simulink model "nonlineardtm"  (R2018b)
settings: configuration reference "Physics" (kept outside this file)
model workspace (MAT data in the model file):
  MCOS : class17 (value not decoded)
undefined symbols (not defined in the file): INIT__initialvalues__Vehicle_InitialPitchAngle, INIT__initialvalues__Vehicle_InitialPitchRate_radps, INIT__initialvalues__Vehicle_InitialVelocity_mps__2, INIT__initialvalues__Vehicle_InitialVelocity_mps__3, INIT__initialvalues__Vehicle_InitialYawAngle, INIT__initialvalues__Vehicle_InitialYawRate_radps, tireFL__INERTIAL__m_Wheel_kg, tireFL__SCALING__LCX, tireFL__SCALING__LCY, tireFL__SCALING__LCZ, tireFL__SCALING__LEX, tireFL__SCALING__LEY, tireFL__SCALING__LFZO, tireFL__SCALING__LGAY, tireFL__SCALING__LGAZ, tireFL__SCALING__LHX, tireFL__SCALING__LHY, tireFL__SCALING__LKX, tireFL__SCALING__LKY, tireFL__SCALING__LMPHI, tireFL__SCALING__LMUV, tireFL__SCALING__LMX, tireFL__SCALING__LMY, tireFL__SCALING__LRES, tireFL__SCALING__LS, tireFL__SCALING__LTR, tireFL__SCALING__LVMX, tireFL__SCALING__LVX, tireFL__SCALING__LVY, tireFL__SCALING__LVYKA, tireFL__SCALING__LXAL, tireFL__SCALING__LYKA, tireFR__INERTIAL__m_Wheel_kg, tireFR__SCALING__LCX, tireFR__SCALING__LCY, tireFR__SCALING__LCZ, tireFR__SCALING__LEX, tireFR__SCALING__LEY, tireFR__SCALING__LFZO, tireFR__SCALING__LGAY, tireFR__SCALING__LGAZ, tireFR__SCALING__LHX, tireFR__SCALING__LHY, tireFR__SCALING__LKX, tireFR__SCALING__LKY, tireFR__SCALING__LMPHI, tireFR__SCALING__LMUV, tireFR__SCALING__LMX, tireFR__SCALING__LMY, tireFR__SCALING__LRES, tireFR__SCALING__LS, tireFR__SCALING__LTR, tireFR__SCALING__LVMX, tireFR__SCALING__LVX, tireFR__SCALING__LVY, tireFR__SCALING__LVYKA, tireFR__SCALING__LXAL, tireFR__SCALING__LYKA, tireRL__INERTIAL__m_Wheel_kg, tireRL__SCALING__LCX ... (+71)
libraries: vehdynlibtire_TUM x4, vehdynlibsuspension x2, vrlib x1, vehdynlibeom_TUM x1
(part 4 of 5)

== system nonlineardtm/Nonlinear Dual Track Model/Computation Chassis Coordinate System ==
  TransformationAngles : Inport
  Transformation : Inport  Port=2
  Wheel : Inport  Port=3
  Add : Sum
  Bus Creator : BusCreator  Inputs=10
  Bus Selector2 : BusSelector  OutputSignals=r_I_IRji_m
  Bus Selector3 : BusSelector  OutputSignals=A_F_I
  Bus Selector4 : BusSelector  OutputSignals=chi_IO_rad
  Derivative{,1..3} (4 alike) : Derivative
  Gain : Gain  Gain=1/2
  Gain1 : Gain  Gain=1/2
  Matrix Multiply{,1..3} (4 alike) : Product  Multiplication=Matrix(*)
  Reshape : Reshape  OutputDimensionality=Column vector (2-D)
  Selector : Selector  NumberOfDimensions=2  InputPortWidth=3  IndexOptions=Select all,Index vector (dialog)  Indices=[3 4],[4]  OutputSizes=1,1
  Selector1 : Selector  NumberOfDimensions=2  InputPortWidth=3  IndexOptions=Select all,Index vector (dialog)  Indices=[3 4],[3]  OutputSizes=1,1
  Signal Conversion3 : SignalConversion  OverrideOpt=off
  Signal Specification{,1..9} (10 alike) : SignalSpecification  Dimensions=[3,1]
  Chassis : Outport
  wires:
  Wheel/1 -> Bus Selector2/1
  Transformation/1 -> Bus Selector3/1
  TransformationAngles/1 -> Bus Selector4/1
  Bus Selector4/1 -> Signal Conversion3/1  "<chi_IO_rad>"
  Derivative/1 -> Matrix Multiply2/2, Signal Specification4/1, Derivative1/1
  Derivative1/1 -> Matrix Multiply3/2, Signal Specification5/1
  Signal Conversion3/1 -> Signal Specification3/1, Derivative/1
  Bus Creator/1 -> Chassis/1
  Derivative2/1 -> Matrix Multiply/2, Signal Specification1/1, Derivative3/1
  Bus Selector2/1 -> Selector/1, Selector1/1  "<r_I_IRji_m>"
  Selector/1 -> Gain1/1
  Add/1 -> Reshape/1
  Reshape/1 -> Derivative2/1, Signal Specification/1
  Derivative3/1 -> Matrix Multiply1/2, Signal Specification2/1
  Signal Specification/1 -> Bus Creator/1  "r_I_IF_m"
  Signal Specification1/1 -> Bus Creator/2  "v_I_IF_mps"
  Signal Specification2/1 -> Bus Creator/3  "a_I_IF_mps2"
  Signal Specification3/1 -> Bus Creator/4  "phi_IF_rad"
  Signal Specification4/1 -> Bus Creator/5  "omega_I_IF_radps"
  Signal Specification5/1 -> Bus Creator/6  "alpha_I_IF_radps2"
  Selector1/1 -> Gain/1
  Gain/1 -> Add/1
  Gain1/1 -> Add/2
  Signal Specification6/1 -> Bus Creator/7  "v_F_IF_mps"
  Signal Specification7/1 -> Bus Creator/8  "a_F_IF_mps2"
  Signal Specification8/1 -> Bus Creator/9  "omega_F_IF_radps"
  Signal Specification9/1 -> Bus Creator/10  "alpha_F_IF_radps2"
  Matrix Multiply/1 -> Signal Specification6/1
  Matrix Multiply1/1 -> Signal Specification7/1
  Matrix Multiply2/1 -> Signal Specification8/1
  Matrix Multiply3/1 -> Signal Specification9/1
  Bus Selector3/1 -> Matrix Multiply/1, Matrix Multiply1/1, Matrix Multiply2/1, Matrix Multiply3/1  "<A_F_I>"

== system nonlineardtm/Nonlinear Dual Track Model/Rearrange Force Bus ==
  VehicleForces : Inport
  SuspensionForces : Inport  Port=2
  TireForces : Inport  Port=3
  Bus Creator : BusCreator  Inputs=13
  Bus Selector : BusSelector  OutputSignals=F_K_sum_N,T_K_sum_Nm,F_K_d_N,T_K_d_Nm,F_K_g_N
  Bus Selector1 : BusSelector  OutputSignals=F_K_Aji_N,T_K_Aji_Nm,F_F_Aji_N,T_F_Aji_Nm
  Bus Selector2 : BusSelector  OutputSignals=F_F_Tji_N,T_F_Tji_Nm,F_Tji_Tji_N,T_Tji_Tji_Nm
  Force : Outport
  wires:
  VehicleForces/1 -> Bus Selector/1
  SuspensionForces/1 -> Bus Selector1/1
  TireForces/1 -> Bus Selector2/1
  Bus Selector/1 -> Bus Creator/1  "<F_K_sum_N>"
  Bus Selector2/4 -> Bus Creator/13  "<T_Tji_Tji_Nm>"
  Bus Selector/2 -> Bus Creator/2  "<T_K_sum_Nm>"
  Bus Selector/3 -> Bus Creator/3  "<F_K_d_N>"
  Bus Selector/4 -> Bus Creator/4  "<T_K_d_Nm>"
  Bus Selector/5 -> Bus Creator/5  "<F_K_g_N>"
  Bus Selector1/1 -> Bus Creator/6  "<F_K_Aji_N>"
  Bus Selector1/2 -> Bus Creator/7  "<T_K_Aji_Nm>"
  Bus Selector1/3 -> Bus Creator/8  "<F_F_Aji_N>"
  Bus Selector1/4 -> Bus Creator/9  "<T_F_Aji_Nm>"
  Bus Selector2/1 -> Bus Creator/10  "<F_F_Tji_N>"
  Bus Selector2/2 -> Bus Creator/11  "<T_F_Tji_Nm>"
  Bus Selector2/3 -> Bus Creator/12  "<F_Tji_Tji_N>"
  Bus Creator/1 -> Force/1

== system nonlineardtm/Nonlinear Dual Track Model/Rotation RoadVerticalDisplacement InertialFrame to TireFixed ==
  z_I_Ground_m : Inport
  Gain1 : Gain  Gain=-1
  z_Tji_Ground_m : Outport
  wires:
  Gain1/1 -> z_Tji_Ground_m/1
  z_I_Ground_m/1 -> Gain1/1

== system nonlineardtm/Nonlinear Dual Track Model/Rotation Vertical Position TireFixed to RearAxleFixed z-down ==
  rz_Tji_Rji_m : Inport
  Gain1 : Gain  Gain=-1
  rz_F_Rji_m : Outport
  wires:
  rz_Tji_Rji_m/1 -> Gain1/1
  Gain1/1 -> rz_F_Rji_m/1

== system nonlineardtm/Nonlinear Dual Track Model/Rotation Vertical Velocity TireFixed to RearAxleFixed z-down ==
  vz_Tji_Rji_mps : Inport
  Gain1 : Gain  Gain=-1
  vz_F_Rji_mps : Outport
  wires:
  vz_Tji_Rji_mps/1 -> Gain1/1
  Gain1/1 -> vz_F_Rji_mps/1

== system nonlineardtm/Nonlinear Dual Track Model/Subsystem ==
  r_F_IAji_m : Inport
  v_F_IAji_mps : Inport  Port=2
  delta_ji_rad : Inport  Port=3
  rz_F_IRji_m : Inport  Port=4
  re_Rji_m : Inport  Port=5
  vz_F_IRji_mps : Inport  Port=6
  F_F_Tji_N : Inport  Port=7
  T_F_Tji_Nm : Inport  Port=8
  Selector3 : Selector  NumberOfDimensions=2  InputPortWidth=1  IndexOptions=Index vector (dialog),Select all  Indices=[2],1  OutputSizes=1,1
  Selector38 : Selector  InputPortWidth=4  IndexOptions=Index vector (dialog)  Indices=[1 2]  OutputSizes=1
  Selector6 : Selector  NumberOfDimensions=2  InputPortWidth=1  IndexOptions=Index vector (dialog),Select all  Indices=[1],1  OutputSizes=1,1
  Signal Conversion{1..7,16} (8 alike) : SignalConversion  OverrideOpt=off
  Signal Specification1 : SignalSpecification  Dimensions=[3,4]
  Signal Specification{2,4,6..8} (5 alike) : SignalSpecification  Dimensions=[1,4]
  Signal Specification3 : SignalSpecification  Dimensions=[3,4]
  Signal Specification5 : SignalSpecification  Dimensions=[3,4]
  VehP [3x4] : Outport
  VehV [3x4] : Outport  Port=2
  StrgAngF [1x2] : Outport  Port=3
  WhlPz [1x4] : Outport  Port=4
  WhlRe [1x4] : Outport  Port=5
  WhlVz [1x4] : Outport  Port=6
  WhlFx [1x4] : Outport  Port=7
  WhlFy [1x4] : Outport  Port=8
  WhlM [3x4] : Outport  Port=9
  wires:
  r_F_IAji_m/1 -> Signal Conversion16/1
  v_F_IAji_mps/1 -> Signal Conversion1/1
  delta_ji_rad/1 -> Signal Conversion2/1
  Signal Specification3/1 -> VehP [3x4]/1
  Signal Specification1/1 -> VehV [3x4]/1
  F_F_Tji_N/1 -> Signal Conversion6/1
  Selector6/1 -> Signal Specification2/1
  Selector3/1 -> Signal Specification4/1
  Signal Specification2/1 -> WhlFx [1x4]/1
  Signal Specification4/1 -> WhlFy [1x4]/1
  Selector38/1 -> StrgAngF [1x2]/1
  T_F_Tji_Nm/1 -> Signal Conversion7/1
  Signal Specification5/1 -> WhlM [3x4]/1
  Signal Specification8/1 -> WhlPz [1x4]/1
  Signal Specification7/1 -> WhlRe [1x4]/1
  Signal Specification6/1 -> WhlVz [1x4]/1
  vz_F_IRji_mps/1 -> Signal Conversion5/1
  re_Rji_m/1 -> Signal Conversion4/1
  rz_F_IRji_m/1 -> Signal Conversion3/1
  Signal Conversion16/1 -> Signal Specification3/1
  Signal Conversion1/1 -> Signal Specification1/1
  Signal Conversion2/1 -> Selector38/1
  Signal Conversion3/1 -> Signal Specification8/1
  Signal Conversion4/1 -> Signal Specification7/1
  Signal Conversion5/1 -> Signal Specification6/1
  Signal Conversion7/1 -> Signal Specification5/1
  Signal Conversion6/1 -> Selector3/1, Selector6/1

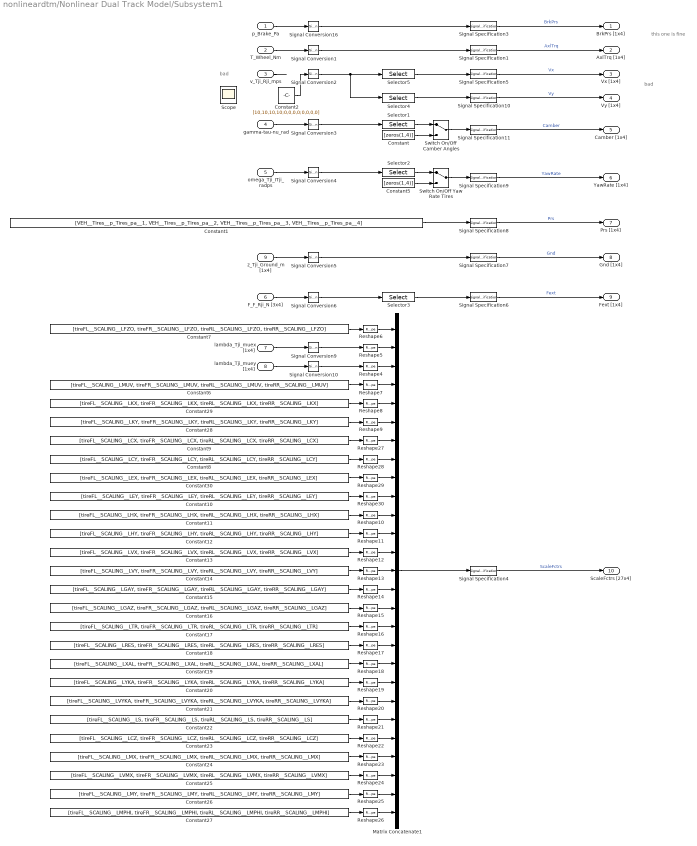
== system nonlineardtm/Nonlinear Dual Track Model/Subsystem1 ==
  note: bad
  note: bad
  note: this one is fine
  p_Brake_Pa : Inport
  T_Wheel_Nm : Inport  Port=2
  v_Tji_Rji_mps : Inport  Port=3
  gamma-tau-nu_rad : Inport  Port=4
  omega_Tji_ITji_radps : Inport  Port=5
  F_F_Rji_N [3x4] : Inport  Port=6
  lambda_Tji_muex [1x4] : Inport  Port=7
  lambda_Tji_muey [1x4] : Inport  Port=8
  z_Tji_Ground_m [1x4] : Inport  Port=9
  Constant : Constant  Value=[zeros(1,4)]
  Constant1 : Constant  Value=[VEH__Tires__p_Tires_pa__1, VEH__Tires__p_Tires_pa__2, VEH__Tires__p_Tires_pa__3, VEH__Tires__p_Tires_pa__4]
  Constant10 : Constant  Value=[tireFL__SCALING__LEY, tireFR__SCALING__LEY, tireRL__SCALING__LEY, tireRR__SCALING__LEY]
  Constant11 : Constant  Value=[tireFL__SCALING__LHX, tireFR__SCALING__LHX, tireRL__SCALING__LHX, tireRR__SCALING__LHX]
  Constant12 : Constant  Value=[tireFL__SCALING__LHY, tireFR__SCALING__LHY, tireRL__SCALING__LHY, tireRR__SCALING__LHY]
  Constant13 : Constant  Value=[tireFL__SCALING__LVX, tireFR__SCALING__LVX, tireRL__SCALING__LVX, tireRR__SCALING__LVX]
  Constant14 : Constant  Value=[tireFL__SCALING__LVY, tireFR__SCALING__LVY, tireRL__SCALING__LVY, tireRR__SCALING__LVY]
  Constant15 : Constant  Value=[tireFL__SCALING__LGAY, tireFR__SCALING__LGAY, tireRL__SCALING__LGAY, tireRR__SCALING__LGAY]
  Constant16 : Constant  Value=[tireFL__SCALING__LGAZ, tireFR__SCALING__LGAZ, tireRL__SCALING__LGAZ, tireRR__SCALING__LGAZ]
  Constant17 : Constant  Value=[tireFL__SCALING__LTR, tireFR__SCALING__LTR, tireRL__SCALING__LTR, tireRR__SCALING__LTR]
  Constant18 : Constant  Value=[tireFL__SCALING__LRES, tireFR__SCALING__LRES, tireRL__SCALING__LRES, tireRR__SCALING__LRES]
  Constant19 : Constant  Value=[tireFL__SCALING__LXAL, tireFR__SCALING__LXAL, tireRL__SCALING__LXAL, tireRR__SCALING__LXAL]
  Constant2 : Constant  Value=[10,10,10,10;0,0,0,0;0,0,0,0]  VectorParams1D=off
  Constant20 : Constant  Value=[tireFL__SCALING__LYKA, tireFR__SCALING__LYKA, tireRL__SCALING__LYKA, tireRR__SCALING__LYKA]
  Constant21 : Constant  Value=[tireFL__SCALING__LVYKA, tireFR__SCALING__LVYKA, tireRL__SCALING__LVYKA, tireRR__SCALING__LVYKA]
  Constant22 : Constant  Value=[tireFL__SCALING__LS, tireFR__SCALING__LS, tireRL__SCALING__LS, tireRR__SCALING__LS]
  Constant23 : Constant  Value=[tireFL__SCALING__LCZ, tireFR__SCALING__LCZ, tireRL__SCALING__LCZ, tireRR__SCALING__LCZ]
  Constant24 : Constant  Value=[tireFL__SCALING__LMX, tireFR__SCALING__LMX, tireRL__SCALING__LMX, tireRR__SCALING__LMX]
  Constant25 : Constant  Value=[tireFL__SCALING__LVMX, tireFR__SCALING__LVMX, tireRL__SCALING__LVMX, tireRR__SCALING__LVMX]
  Constant26 : Constant  Value=[tireFL__SCALING__LMY, tireFR__SCALING__LMY, tireRL__SCALING__LMY, tireRR__SCALING__LMY]
  Constant27 : Constant  Value=[tireFL__SCALING__LMPHI, tireFR__SCALING__LMPHI, tireRL__SCALING__LMPHI, tireRR__SCALING__LMPHI]
  Constant28 : Constant  Value=[tireFL__SCALING__LKY, tireFR__SCALING__LKY, tireRL__SCALING__LKY, tireRR__SCALING__LKY]
  Constant29 : Constant  Value=[tireFL__SCALING__LKX, tireFR__SCALING__LKX, tireRL__SCALING__LKX, tireRR__SCALING__LKX]
  Constant30 : Constant  Value=[tireFL__SCALING__LEX, tireFR__SCALING__LEX, tireRL__SCALING__LEX, tireRR__SCALING__LEX]
  Constant5 : Constant  Value=[zeros(1,4)]
  Constant6 : Constant  Value=[tireFL__SCALING__LMUV, tireFR__SCALING__LMUV, tireRL__SCALING__LMUV, tireRR__SCALING__LMUV]
  Constant7 : Constant  Value=[tireFL__SCALING__LFZO, tireFR__SCALING__LFZO, tireRL__SCALING__LFZO, tireRR__SCALING__LFZO]
  Constant8 : Constant  Value=[tireFL__SCALING__LCY, tireFR__SCALING__LCY, tireRL__SCALING__LCY, tireRR__SCALING__LCY]
  Constant9 : Constant  Value=[tireFL__SCALING__LCX, tireFR__SCALING__LCX, tireRL__SCALING__LCX, tireRR__SCALING__LCX]
  Matrix Concatenate1 : Concatenate  NumInputs=27  Mode=Multidimensional array
  Reshape{4..30} (27 alike) : Reshape  OutputDimensionality=Row vector (2-D)
  Scope : Scope
  Selector1 : Selector  NumberOfDimensions=2  InputPortWidth=3  IndexOptions=Index vector (dialog),Select all  Indices=1,1  OutputSizes=1,1
  Selector2 : Selector  NumberOfDimensions=2  InputPortWidth=3  IndexOptions=Index vector (dialog),Select all  Indices=3,1  OutputSizes=1,1
  Selector3 : Selector  NumberOfDimensions=2  InputPortWidth=3  IndexOptions=Index vector (dialog),Select all  Indices=3,1  OutputSizes=1,1
  Selector4 : Selector  NumberOfDimensions=2  InputPortWidth=1  IndexOptions=Index vector (dialog),Select all  Indices=[2],1  OutputSizes=1,1
  Selector5 : Selector  NumberOfDimensions=2  InputPortWidth=1  IndexOptions=Index vector (dialog),Select all  Indices=[1],1  OutputSizes=1,1
  Signal Conversion{1..6,9..10,16} (9 alike) : SignalConversion  OverrideOpt=off
  Signal Specification{1,3,5..11} (9 alike) : SignalSpecification  Dimensions=[1,4]
  Signal Specification4 : SignalSpecification  Dimensions=[27,4]
  Switch On/Off Camber Angles : ManualSwitch
  Switch On/Off Yaw Rate Tires : ManualSwitch
  BrkPrs [1x4] : Outport
  AxlTrq [1x4] : Outport  Port=2
  Vx [1x4] : Outport  Port=3
  Vy [1x4] : Outport  Port=4
  Camber [1x4] : Outport  Port=5
  YawRate [1x4] : Outport  Port=6
  Prs [1x4] : Outport  Port=7
  Gnd [1x4] : Outport  Port=8
  Fext [1x4] : Outport  Port=9
  ScaleFctrs [27x4] : Outport  Port=10
  wires:
  Signal Specification9/1 -> YawRate [1x4]/1  "YawRate"
  Signal Specification1/1 -> AxlTrq [1x4]/1  "AxlTrq"
  Signal Specification4/1 -> ScaleFctrs [27x4]/1  "ScaleFctrs"
  Signal Specification8/1 -> Prs [1x4]/1  "Prs"
  Signal Specification7/1 -> Gnd [1x4]/1  "Gnd"
  Signal Specification6/1 -> Fext [1x4]/1  "Fext"
  Signal Specification5/1 -> Vx [1x4]/1  "Vx"
  Signal Specification10/1 -> Vy [1x4]/1  "Vy"
  Constant1/1 -> Signal Specification8/1
  Signal Specification11/1 -> Camber [1x4]/1  "Camber"
  Selector1/1 -> Switch On/Off Camber Angles/1
  Switch On/Off Camber Angles/1 -> Signal Specification11/1
  Constant/1 -> Switch On/Off Camber Angles/2
  Constant5/1 -> Switch On/Off Yaw Rate Tires/2
  Switch On/Off Yaw Rate Tires/1 -> Signal Specification9/1
  Selector2/1 -> Switch On/Off Yaw Rate Tires/1
  p_Brake_Pa/1 -> Signal Conversion16/1
  T_Wheel_Nm/1 -> Signal Conversion1/1
  gamma-tau-nu_rad/1 -> Signal Conversion3/1
  omega_Tji_ITji_radps/1 -> Signal Conversion4/1
  z_Tji_Ground_m [1x4]/1 -> Signal Conversion5/1
  F_F_Rji_N [3x4]/1 -> Signal Conversion6/1
  Signal Specification3/1 -> BrkPrs [1x4]/1  "BrkPrs"
  Signal Conversion16/1 -> Signal Specification3/1
  Signal Conversion1/1 -> Signal Specification1/1
  Signal Conversion3/1 -> Selector1/1
  Signal Conversion5/1 -> Signal Specification7/1
  Signal Conversion2/1 -> Selector4/1, Selector5/1
  Signal Conversion4/1 -> Selector2/1
  Signal Conversion6/1 -> Selector3/1
  Selector5/1 -> Signal Specification5/1
  Selector4/1 -> Signal Specification10/1
  Selector3/1 -> Signal Specification6/1
  lambda_Tji_muey [1x4]/1 -> Signal Conversion10/1
  lambda_Tji_muex [1x4]/1 -> Signal Conversion9/1
  Constant7/1 -> Reshape6/1
  Reshape5/1 -> Matrix Concatenate1/2
  Reshape27/1 -> Matrix Concatenate1/7
  Constant28/1 -> Reshape9/1
  Constant13/1 -> Reshape12/1
  Constant9/1 -> Reshape27/1
  Reshape7/1 -> Matrix Concatenate1/4
  Reshape16/1 -> Matrix Concatenate1/17
  Constant21/1 -> Reshape20/1
  Reshape11/1 -> Matrix Concatenate1/12
  Reshape9/1 -> Matrix Concatenate1/6
  Signal Conversion9/1 -> Reshape5/1
  Reshape17/1 -> Matrix Concatenate1/18
  Reshape25/1 -> Matrix Concatenate1/26
  Reshape29/1 -> Matrix Concatenate1/9
  Constant29/1 -> Reshape8/1
  Constant12/1 -> Reshape11/1
  Constant30/1 -> Reshape29/1
  Signal Conversion10/1 -> Reshape4/1
  Reshape24/1 -> Matrix Concatenate1/25
  Constant20/1 -> Reshape19/1
  Constant6/1 -> Reshape7/1
  Constant15/1 -> Reshape14/1
  Constant26/1 -> Reshape25/1
  Reshape12/1 -> Matrix Concatenate1/13
  Constant11/1 -> Reshape10/1
  Constant16/1 -> Reshape15/1
  Constant23/1 -> Reshape22/1
  Reshape15/1 -> Matrix Concatenate1/16
  Reshape10/1 -> Matrix Concatenate1/11
  Reshape18/1 -> Matrix Concatenate1/19
  Matrix Concatenate1/1 -> Signal Specification4/1
  Constant22/1 -> Reshape21/1
  Reshape6/1 -> Matrix Concatenate1/1
  Constant10/1 -> Reshape30/1
  Reshape26/1 -> Matrix Concatenate1/27
  Reshape14/1 -> Matrix Concatenate1/15
  Reshape4/1 -> Matrix Concatenate1/3
  Reshape22/1 -> Matrix Concatenate1/23
  Reshape20/1 -> Matrix Concatenate1/21
  Constant19/1 -> Reshape18/1
  Reshape8/1 -> Matrix Concatenate1/5
  Constant18/1 -> Reshape17/1
  Constant17/1 -> Reshape16/1
  Reshape19/1 -> Matrix Concatenate1/20
  Reshape30/1 -> Matrix Concatenate1/10
  Constant27/1 -> Reshape26/1
  Reshape13/1 -> Matrix Concatenate1/14
  Reshape21/1 -> Matrix Concatenate1/22
  Constant14/1 -> Reshape13/1
  Reshape28/1 -> Matrix Concatenate1/8
  Reshape23/1 -> Matrix Concatenate1/24
  Constant24/1 -> Reshape23/1
  Constant25/1 -> Reshape24/1
  Constant8/1 -> Reshape28/1
  v_Tji_Rji_mps/1 -> ?
  Constant2/1 -> Signal Conversion2/1

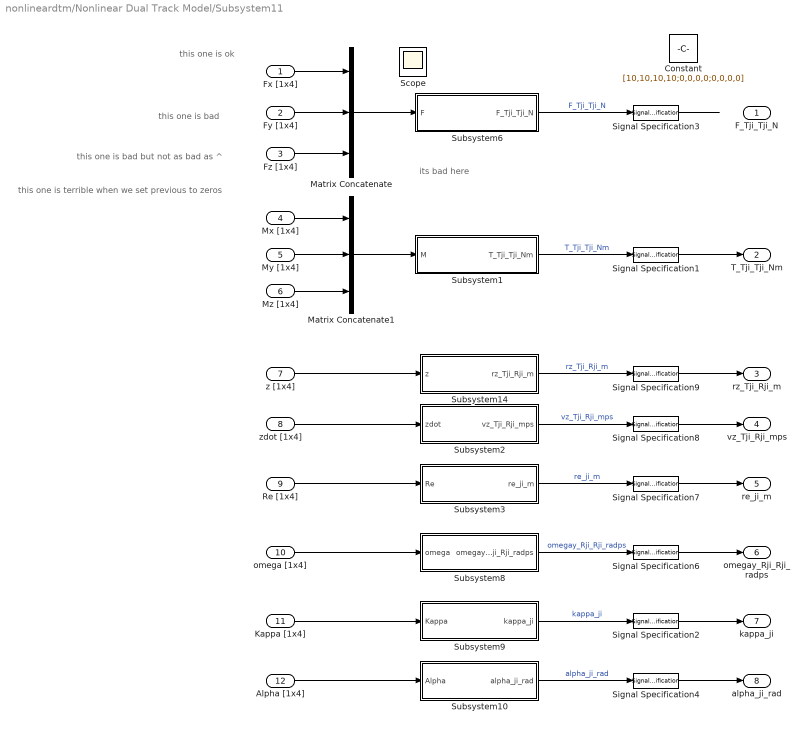
== system nonlineardtm/Nonlinear Dual Track Model/Subsystem11 ==
  note: this one is terrible when we set previous to zeros
  note: this one is bad but not as bad as ^
  note: this one is bad
  note: its bad here
  note: this one is ok
  Fx [1x4] : Inport
  Fy [1x4] : Inport  Port=2
  Fz [1x4] : Inport  Port=3
  Mx [1x4] : Inport  Port=4
  My [1x4] : Inport  Port=5
  Mz [1x4] : Inport  Port=6
  z [1x4] : Inport  Port=7
  zdot [1x4] : Inport  Port=8
  Re [1x4] : Inport  Port=9
  omega [1x4] : Inport  Port=10
  Kappa [1x4] : Inport  Port=11
  Alpha [1x4] : Inport  Port=12
  Constant : Constant  Value=[10,10,10,10;0,0,0,0;0,0,0,0]
  Matrix Concatenate : Concatenate  NumInputs=3  Mode=Multidimensional array
  Matrix Concatenate1 : Concatenate  NumInputs=3  Mode=Multidimensional array
  Scope : Scope
  Signal Specification1 : SignalSpecification  Dimensions=[3,4]
  Signal Specification{2,4,6..9} (6 alike) : SignalSpecification  Dimensions=[1,4]
  Signal Specification3 : SignalSpecification  Dimensions=[3,4]
  Subsystem1 : Subsystem
  Subsystem10 : Subsystem
  Subsystem14 : Subsystem
  Subsystem2 : Subsystem
  Subsystem3 : Subsystem
  Subsystem6 : Subsystem
  Subsystem8 : Subsystem
  Subsystem9 : Subsystem
  F_Tji_Tji_N : Outport
  T_Tji_Tji_Nm : Outport  Port=2
  rz_Tji_Rji_m : Outport  Port=3
  vz_Tji_Rji_mps : Outport  Port=4
  re_ji_m : Outport  Port=5
  omegay_Rji_Rji_radps : Outport  Port=6
  kappa_ji : Outport  Port=7
  alpha_ji_rad : Outport  Port=8
  wires:
  Signal Specification6/1 -> omegay_Rji_Rji_radps/1
  Signal Specification7/1 -> re_ji_m/1
  Signal Specification8/1 -> vz_Tji_Rji_mps/1
  Signal Specification4/1 -> alpha_ji_rad/1
  Signal Specification2/1 -> kappa_ji/1
  Signal Specification1/1 -> T_Tji_Tji_Nm/1
  Signal Specification3/1 -> ?
  Mx [1x4]/1 -> Matrix Concatenate1/1
  Subsystem14/1(rz_Tji_Rji_m) -> Signal Specification9/1  "rz_Tji_Rji_m"
  Fz [1x4]/1 -> Matrix Concatenate/3
  Mz [1x4]/1 -> Matrix Concatenate1/3
  My [1x4]/1 -> Matrix Concatenate1/2
  Fy [1x4]/1 -> Matrix Concatenate/2
  Fx [1x4]/1 -> Matrix Concatenate/1
  Signal Specification9/1 -> rz_Tji_Rji_m/1
  z [1x4]/1 -> Subsystem14/1(z)
  zdot [1x4]/1 -> Subsystem2/1(zdot)
  Re [1x4]/1 -> Subsystem3/1(Re)
  omega [1x4]/1 -> Subsystem8/1(omega)
  Kappa [1x4]/1 -> Subsystem9/1(Kappa)
  Alpha [1x4]/1 -> Subsystem10/1(Alpha)
  Subsystem2/1(vz_Tji_Rji_mps) -> Signal Specification8/1  "vz_Tji_Rji_mps"
  Subsystem3/1(re_ji_m) -> Signal Specification7/1  "re_ji_m"
  Subsystem8/1(omegay_Rji_Rji_radps) -> Signal Specification6/1  "omegay_Rji_Rji_radps"
  Subsystem9/1(kappa_ji) -> Signal Specification2/1  "kappa_ji"
  Subsystem10/1(alpha_ji_rad) -> Signal Specification4/1  "alpha_ji_rad"
  Subsystem1/1(T_Tji_Tji_Nm) -> Signal Specification1/1  "T_Tji_Tji_Nm"
  Subsystem6/1(F_Tji_Tji_N) -> Signal Specification3/1  "F_Tji_Tji_N"
  Matrix Concatenate1/1 -> Subsystem1/1(M)
  Matrix Concatenate/1 -> Subsystem6/1(F)

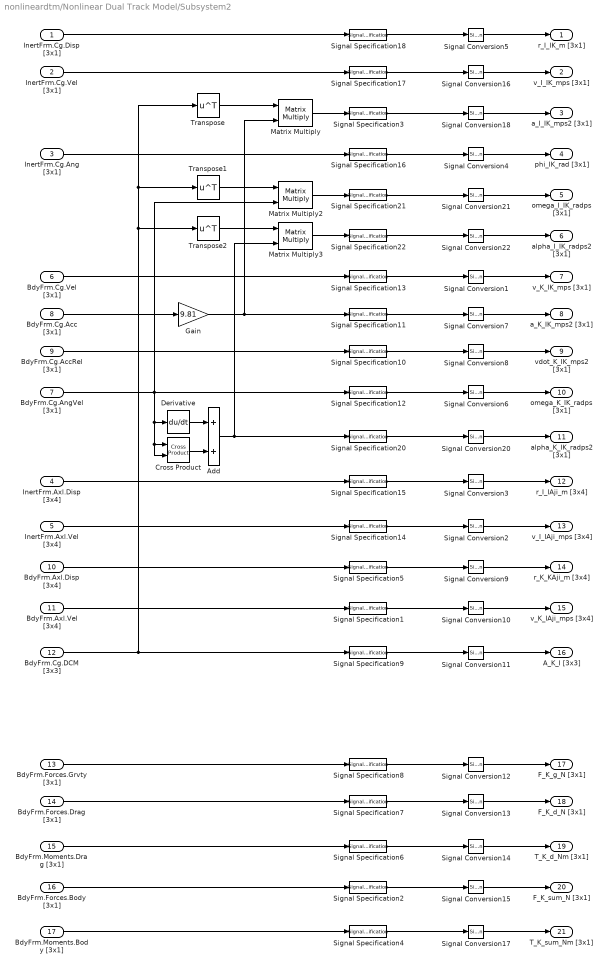
== system nonlineardtm/Nonlinear Dual Track Model/Subsystem2 ==
  InertFrm.Cg.Disp [3x1] : Inport
  InertFrm.Cg.Vel [3x1] : Inport  Port=2
  InertFrm.Cg.Ang [3x1] : Inport  Port=3
  InertFrm.Axl.Disp [3x4] : Inport  Port=4
  InertFrm.Axl.Vel [3x4] : Inport  Port=5
  BdyFrm.Cg.Vel [3x1] : Inport  Port=6
  BdyFrm.Cg.AngVel [3x1] : Inport  Port=7
  BdyFrm.Cg.Acc [3x1] : Inport  Port=8
  BdyFrm.Cg.AccRel [3x1] : Inport  Port=9
  BdyFrm.Axl.Disp [3x4] : Inport  Port=10
  BdyFrm.Axl.Vel [3x4] : Inport  Port=11
  BdyFrm.Cg.DCM [3x3] : Inport  Port=12
  BdyFrm.Forces.Grvty [3x1] : Inport  Port=13
  BdyFrm.Forces.Drag [3x1] : Inport  Port=14
  BdyFrm.Moments.Drag [3x1] : Inport  Port=15
  BdyFrm.Forces.Body [3x1] : Inport  Port=16
  BdyFrm.Moments.Body [3x1] : Inport  Port=17
  Add : Sum
  Cross Product : vrlib/Utilities/Cross Product
      settings: SourceProductBaseCode=VR
  Derivative : Derivative
  Gain : Gain  Gain=9.81
  Matrix Multiply : Product  Multiplication=Matrix(*)
  Matrix Multiply2 : Product  Multiplication=Matrix(*)
  Matrix Multiply3 : Product  Multiplication=Matrix(*)
  Signal Conversion{1..18,20..22} (21 alike) : SignalConversion  OverrideOpt=off
  Signal Specification{1,5,14..15} (4 alike) : SignalSpecification  Dimensions=[3,4]
  Signal Specification{2..4,6..8,10..13,16..18,20..22} (16 alike) : SignalSpecification  Dimensions=[3,1]
  Signal Specification9 : SignalSpecification  Dimensions=[3,3]
  Transpose : Math  Operator=transpose  SaturateOnIntegerOverflow=on
  Transpose1 : Math  Operator=transpose  SaturateOnIntegerOverflow=on
  Transpose2 : Math  Operator=transpose  SaturateOnIntegerOverflow=on
  r_I_IK_m [3x1] : Outport
  v_I_IK_mps [3x1] : Outport  Port=2
  a_I_IK_mps2 [3x1] : Outport  Port=3
  phi_IK_rad [3x1] : Outport  Port=4
  omega_I_IK_radps [3x1] : Outport  Port=5
  alpha_I_IK_radps2 [3x1] : Outport  Port=6
  v_K_IK_mps [3x1] : Outport  Port=7
  a_K_IK_mps2 [3x1] : Outport  Port=8
  vdot_K_IK_mps2 [3x1] : Outport  Port=9
  omega_K_IK_radps [3x1] : Outport  Port=10
  alpha_K_IK_radps2 [3x1] : Outport  Port=11
  r_I_IAji_m [3x4] : Outport  Port=12
  v_I_IAji_mps [3x4] : Outport  Port=13
  r_K_KAji_m [3x4] : Outport  Port=14
  v_K_IAji_mps [3x4] : Outport  Port=15
  A_K_I [3x3] : Outport  Port=16
  F_K_g_N [3x1] : Outport  Port=17
  F_K_d_N [3x1] : Outport  Port=18
  T_K_d_Nm [3x1] : Outport  Port=19
  F_K_sum_N [3x1] : Outport  Port=20
  T_K_sum_Nm [3x1] : Outport  Port=21
  wires:
  Signal Specification5/1 -> Signal Conversion9/1
  Signal Specification11/1 -> Signal Conversion7/1
  Signal Specification7/1 -> Signal Conversion13/1
  Signal Specification16/1 -> Signal Conversion4/1
  Signal Specification8/1 -> Signal Conversion12/1
  Signal Specification6/1 -> Signal Conversion14/1
  Signal Specification12/1 -> Signal Conversion6/1
  Signal Specification1/1 -> Signal Conversion10/1
  Signal Specification9/1 -> Signal Conversion11/1
  Signal Specification15/1 -> Signal Conversion3/1
  Signal Specification18/1 -> Signal Conversion5/1
  Signal Specification4/1 -> Signal Conversion17/1
  Signal Specification13/1 -> Signal Conversion1/1
  Signal Specification10/1 -> Signal Conversion8/1
  Signal Specification14/1 -> Signal Conversion2/1
  Signal Specification2/1 -> Signal Conversion15/1
  Signal Specification17/1 -> Signal Conversion16/1
  BdyFrm.Cg.Acc [3x1]/1 -> Gain/1
  InertFrm.Cg.Disp [3x1]/1 -> Signal Specification18/1
  InertFrm.Cg.Vel [3x1]/1 -> Signal Specification17/1
  InertFrm.Cg.Ang [3x1]/1 -> Signal Specification16/1
  InertFrm.Axl.Disp [3x4]/1 -> Signal Specification15/1
  InertFrm.Axl.Vel [3x4]/1 -> Signal Specification14/1
  BdyFrm.Cg.Vel [3x1]/1 -> Signal Specification13/1
  BdyFrm.Cg.AngVel [3x1]/1 -> Cross Product/2, Cross Product/1, Derivative/1, Matrix Multiply2/2, Signal Specification12/1
  Gain/1 -> Signal Specification11/1, Matrix Multiply/2
  BdyFrm.Cg.AccRel [3x1]/1 -> Signal Specification10/1
  BdyFrm.Axl.Disp [3x4]/1 -> Signal Specification5/1
  BdyFrm.Axl.Vel [3x4]/1 -> Signal Specification1/1
  BdyFrm.Cg.DCM [3x3]/1 -> Signal Specification9/1, Transpose1/1, Transpose/1, Transpose2/1
  BdyFrm.Forces.Grvty [3x1]/1 -> Signal Specification8/1
  BdyFrm.Forces.Drag [3x1]/1 -> Signal Specification7/1
  BdyFrm.Moments.Drag [3x1]/1 -> Signal Specification6/1
  BdyFrm.Forces.Body [3x1]/1 -> Signal Specification2/1
  BdyFrm.Moments.Body [3x1]/1 -> Signal Specification4/1
  Signal Conversion16/1 -> v_I_IK_mps [3x1]/1
  Signal Conversion5/1 -> r_I_IK_m [3x1]/1
  Signal Conversion4/1 -> phi_IK_rad [3x1]/1
  Signal Conversion3/1 -> r_I_IAji_m [3x4]/1
  Signal Conversion2/1 -> v_I_IAji_mps [3x4]/1
  Signal Conversion1/1 -> v_K_IK_mps [3x1]/1
  Signal Conversion6/1 -> omega_K_IK_radps [3x1]/1
  Signal Conversion7/1 -> a_K_IK_mps2 [3x1]/1
  Signal Conversion8/1 -> vdot_K_IK_mps2 [3x1]/1
  Signal Conversion9/1 -> r_K_KAji_m [3x4]/1
  Signal Conversion10/1 -> v_K_IAji_mps [3x4]/1
  Signal Conversion11/1 -> A_K_I [3x3]/1
  Signal Conversion12/1 -> F_K_g_N [3x1]/1
  Signal Conversion13/1 -> F_K_d_N [3x1]/1
  Signal Conversion14/1 -> T_K_d_Nm [3x1]/1
  Signal Conversion15/1 -> F_K_sum_N [3x1]/1
  Signal Conversion17/1 -> T_K_sum_Nm [3x1]/1
  Signal Conversion18/1 -> a_I_IK_mps2 [3x1]/1
  Signal Specification3/1 -> Signal Conversion18/1
  Matrix Multiply/1 -> Signal Specification3/1
  Transpose/1 -> Matrix Multiply/1
  Signal Conversion20/1 -> alpha_K_IK_radps2 [3x1]/1
  Signal Specification20/1 -> Signal Conversion20/1
  Derivative/1 -> Add/1
  Add/1 -> Signal Specification20/1, Matrix Multiply3/2
  Cross Product/1 -> Add/2
  Signal Conversion21/1 -> omega_I_IK_radps [3x1]/1
  Signal Specification21/1 -> Signal Conversion21/1
  Matrix Multiply2/1 -> Signal Specification21/1
  Transpose1/1 -> Matrix Multiply2/1
  Matrix Multiply3/1 -> Signal Specification22/1
  Signal Specification22/1 -> Signal Conversion22/1
  Signal Conversion22/1 -> alpha_I_IK_radps2 [3x1]/1
  Transpose2/1 -> Matrix Multiply3/1

== system nonlineardtm/Nonlinear Dual Track Model/Subsystem3 ==
  F_K_Extern_N : Inport
  T_K_Extern_Nm : Inport  Port=2
  v_I_Wind_mps : Inport  Port=3
  F_K_Aji_N : Inport  Port=4
  T_K_Aji_Nm : Inport  Port=5
  Signal Conversion{1..4,16} (5 alike) : SignalConversion  OverrideOpt=off
  Signal Specification1 : SignalSpecification  Dimensions=[3,1]
  Signal Specification2 : SignalSpecification  Dimensions=[3,1]
  Signal Specification3 : SignalSpecification  Dimensions=[3,1]
  Signal Specification7 : SignalSpecification  Dimensions=[3,4]
  Signal Specification8 : SignalSpecification  Dimensions=[3,4]
  FExt [3x1] : Outport
  MExt [3x1] : Outport  Port=2
  WindXYZ [3x1] : Outport  Port=3
  FSusp [3x4] : Outport  Port=4
  MSusp [3x4] : Outport  Port=5
  wires:
  v_I_Wind_mps/1 -> Signal Specification2/1
  Signal Specification2/1 -> Signal Conversion2/1
  T_K_Aji_Nm/1 -> Signal Specification8/1
  F_K_Aji_N/1 -> Signal Specification7/1
  T_K_Extern_Nm/1 -> Signal Specification1/1
  F_K_Extern_N/1 -> Signal Specification3/1
  Signal Conversion4/1 -> MSusp [3x4]/1
  Signal Conversion3/1 -> FSusp [3x4]/1
  Signal Conversion1/1 -> MExt [3x1]/1
  Signal Conversion16/1 -> FExt [3x1]/1
  Signal Specification7/1 -> Signal Conversion3/1
  Signal Specification8/1 -> Signal Conversion4/1
  Signal Conversion2/1 -> WindXYZ [3x1]/1
  Signal Specification1/1 -> Signal Conversion1/1
  Signal Specification3/1 -> Signal Conversion16/1

== system nonlineardtm/Nonlinear Dual Track Model/Subsystem4 ==
  VehF [3x4] : Inport
  VehM [3x4] : Inport  Port=2
  WhlF [3x4] : Inport  Port=3
  WhlV [3x4] : Inport  Port=4
  WhlAng [3x4] : Inport  Port=5
  SuspH [1x4] : Inport  Port=6
  Signal Conversion{1..5,16} (6 alike) : SignalConversion  OverrideOpt=off
  Signal Specification{1..5} (5 alike) : SignalSpecification  Dimensions=[3,4]
  Signal Specification6 : SignalSpecification  Dimensions=[1,4]
  F_F_Aji_N : Outport
  T_F_Aji_Nm : Outport  Port=2
  F_F_Rji_N : Outport  Port=3
  v_F_IRji_mps : Outport  Port=4
  gamma-tau-nu_rad : Outport  Port=5
  h_ji_m : Outport  Port=6
  wires:
  Signal Specification3/1 -> F_F_Aji_N/1
  Signal Specification1/1 -> T_F_Aji_Nm/1
  WhlF [3x4]/1 -> Signal Conversion2/1
  Signal Specification4/1 -> v_F_IRji_mps/1
  Signal Specification5/1 -> gamma-tau-nu_rad/1
  Signal Specification6/1 -> h_ji_m/1
  VehF [3x4]/1 -> Signal Conversion16/1
  VehM [3x4]/1 -> Signal Conversion1/1
  WhlV [3x4]/1 -> Signal Conversion3/1
  WhlAng [3x4]/1 -> Signal Conversion4/1
  SuspH [1x4]/1 -> Signal Conversion5/1
  Signal Specification2/1 -> F_F_Rji_N/1
  Signal Conversion16/1 -> Signal Specification3/1
  Signal Conversion1/1 -> Signal Specification1/1
  Signal Conversion2/1 -> Signal Specification2/1
  Signal Conversion3/1 -> Signal Specification4/1
  Signal Conversion4/1 -> Signal Specification5/1
  Signal Conversion5/1 -> Signal Specification6/1

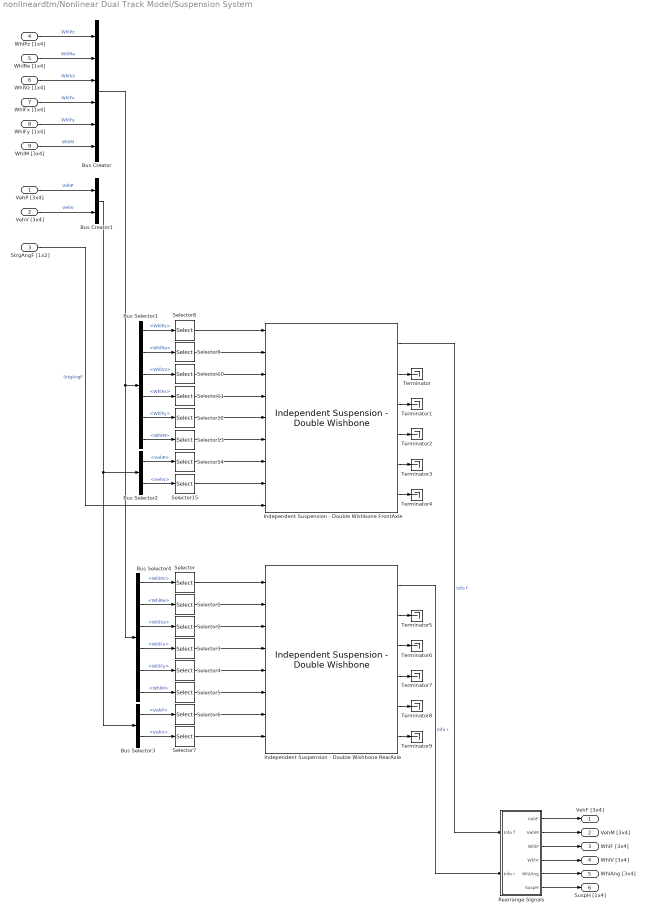
== system nonlineardtm/Nonlinear Dual Track Model/Suspension System ==
  VehP [3x4] : Inport
  VehV [3x4] : Inport  Port=2
  StrgAngF [1x2] : Inport  Port=3
  WhlPz [1x4] : Inport  Port=4
  WhlRe [1x4] : Inport  Port=5
  WhlVz [1x4] : Inport  Port=6
  WhlFx [1x4] : Inport  Port=7
  WhlFy [1x4] : Inport  Port=8
  WhlM [3x4] : Inport  Port=9
  Bus Creator : BusCreator  Inputs=6
  Bus Creator1 : BusCreator  Inputs=2
  Bus Selector1 : BusSelector  OutputSignals=WhlPz,WhlRe,WhlVz,WhlFx,WhlFy,WhlM
  Bus Selector2 : BusSelector  OutputSignals=VehP,VehV
  Bus Selector3 : BusSelector  OutputSignals=VehP,VehV
  Bus Selector4 : BusSelector  OutputSignals=WhlPz,WhlRe,WhlVz,WhlFx,WhlFy,WhlM
  Independent Suspension - Double Wishbone FrontAxle : vehdynlibsuspension/Independent Suspension - Double Wishbone  NumAxl=1  NumTracksByAxl=[2]  StrgEnByAxl=[1]  AntiSwayEnByAxl=[1]  TrackNumVec="[1  2]"  AxleNumVec="[1  1]"  SuspTypesByAxle=[1]  SuspImage=suspdw.png  IdealSuspEn=on  IdealSuspAxles=[1]  Kz=SUS__Compliance__cz_SpringRateFrRe_Npm__1  F0z=SUS__Compliance__F0z_SpringPreloadFrRe_N__1  Cz=SUS__Compliance__Cz_DamperRateFrRe_Nspm__1  Hmax=SUS__Compliance__Hmax_MaxHeightToHardblock_m  Toe=SUS__Kinematics__nu0_ToeATSteerCenterFrRe_rad__1  RollStrgSlp=SUS__Kinematics__k_RollSteerVSHeightFrRe_radpm__1  ToeStrgSlp=SUS__Kinematics__k_ToeVSSteerF  Caster=SUS__Kinematics__k_CasterATSteerCenterF__1  CasterHslp=SUS__Kinematics__k_CasterVSHeightFrRe__1  CasterStrgSlp=SUS__Kinematics__k_CasterVSSteerFrRe  Camber=SUS__Kinematics__k_CamberATSteerCenterF__1  CamberHslp=SUS__Kinematics__k_CamberVSHeightFrRe__1  CamberStrgSlp=SUS__Kinematics__k_CamberVSSteerF  StrgHgtSlp=SUS__Kinematics__k_HeightVSSteerF_mprad  MappedSuspEn=off  MappedSuspAxles="[1  2]"  f_susp_axl_bp=[1 2]  f_susp_dz_bp=[-0.15 -0.14 -0.13 -0.12 -0.11 -0.10 -0.09 -0.08 -0.07 -0.06 -0.05 -0.04 -0.03 -0.02 -0.01 0.00 0.01 0.02 0.03 0.04 0.05 0.06 0.07 0.08 0.09 0.10 0.11 0.12 0.13 0.14 0.15]  f_susp_dzdot_bp=[-0.15 -0.14 -0.13 -0.12 -0.11 -0.10 -0.09 -0.08 -0.07 -0.06 -0.05 -0.04 -0.03 -0.02 -0.01 0.00 0.01 0.02 0.03 0.04 0.05 0.06 0.07 0.08 0.09 0.10 0.11 0.12 0.13 0.14 0.15]  f_susp_fmz=zeros(31,31,61,2,4)  f_susp_geom=zeros(31,61,2,3)  f_susp_strgdelta_bp=[-30,-29,-28,-27,-26,-25,-24,-23,-22,-21,-20,-19,-18,-17,-16,-15,-14,-13,-12,-11,-10,-9,-8,-7,-6,-5,-4,-3,-2,-1,0,1,2,3,4,5,6,7,8,9,10,11,12,13,14,15,16,17,18,19,20,21,22,23,24,25,26,27,28,29,30]  AntiSwayR=SUS__Antisway__r_AntiSwayArmRadiusFrRe_m__1  AntiSwayNtrlAng=SUS__Antisway__phi_AntiSwayNeutralAngleFrRe_rad__1  AntiSwayTrsK=SUS__Antisway__c_AntiSwayTSpringFrRe_Nmprad__1
      settings: SourceProductName=Vehicle Dynamics Blockset  SourceProductBaseCode=VE
  Independent Suspension - Double Wishbone RearAxle : vehdynlibsuspension/Independent Suspension - Double Wishbone  NumAxl=1  NumTracksByAxl=[2]  StrgEnByAxl=[0]  AntiSwayEnByAxl=[1]  TrackNumVec="[1  2]"  AxleNumVec="[1  1]"  SuspTypesByAxle=[1]  SuspImage=suspdw.png  IdealSuspEn=on  IdealSuspAxles=[1]  Kz=SUS__Compliance__cz_SpringRateFrRe_Npm__2  F0z=SUS__Compliance__F0z_SpringPreloadFrRe_N__2  Cz=SUS__Compliance__Cz_DamperRateFrRe_Nspm__2  Hmax=SUS__Compliance__Hmax_MaxHeightToHardblock_m  Toe=SUS__Kinematics__nu0_ToeATSteerCenterFrRe_rad__2  RollStrgSlp=SUS__Kinematics__k_RollSteerVSHeightFrRe_radpm__2  ToeStrgSlp=0  Caster=SUS__Kinematics__k_CasterATSteerCenterF__2  CasterHslp=SUS__Kinematics__k_CasterVSHeightFrRe__2  CasterStrgSlp=0  Camber=SUS__Kinematics__k_CamberATSteerCenterF__2  CamberHslp=SUS__Kinematics__k_CamberVSHeightFrRe__2  CamberStrgSlp=0  StrgHgtSlp=0  MappedSuspEn=off  MappedSuspAxles="[1  2]"  f_susp_axl_bp=[1 2]  f_susp_dz_bp=[-0.15 -0.14 -0.13 -0.12 -0.11 -0.10 -0.09 -0.08 -0.07 -0.06 -0.05 -0.04 -0.03 -0.02 -0.01 0.00 0.01 0.02 0.03 0.04 0.05 0.06 0.07 0.08 0.09 0.10 0.11 0.12 0.13 0.14 0.15]  f_susp_dzdot_bp=[-0.15 -0.14 -0.13 -0.12 -0.11 -0.10 -0.09 -0.08 -0.07 -0.06 -0.05 -0.04 -0.03 -0.02 -0.01 0.00 0.01 0.02 0.03 0.04 0.05 0.06 0.07 0.08 0.09 0.10 0.11 0.12 0.13 0.14 0.15]  f_susp_fmz=zeros(31,31,61,2,4)  f_susp_geom=zeros(31,61,2,3)  f_susp_strgdelta_bp=[-30,-29,-28,-27,-26,-25,-24,-23,-22,-21,-20,-19,-18,-17,-16,-15,-14,-13,-12,-11,-10,-9,-8,-7,-6,-5,-4,-3,-2,-1,0,1,2,3,4,5,6,7,8,9,10,11,12,13,14,15,16,17,18,19,20,21,22,23,24,25,26,27,28,29,30]  AntiSwayR=SUS__Antisway__r_AntiSwayArmRadiusFrRe_m__2  AntiSwayNtrlAng=SUS__Antisway__phi_AntiSwayNeutralAngleFrRe_rad__2  AntiSwayTrsK=SUS__Antisway__c_AntiSwayTSpringFrRe_Nmprad__2
      settings: SourceProductName=Vehicle Dynamics Blockset  SourceProductBaseCode=VE
  Rearrange Signals : Subsystem
  Selector{,1..4} (5 alike) : Selector  InputPortWidth=4  IndexOptions=Index vector (dialog)  Indices=[3 4]  OutputSizes=1
  Selector{8..12} (5 alike) : Selector  InputPortWidth=4  IndexOptions=Index vector (dialog)  Indices=[1 2]  OutputSizes=1
  Selector13 : Selector  NumberOfDimensions=2  InputPortWidth=4  IndexOptions=Select all,Index vector (dialog)  Indices=[1 2],[1 2]  OutputSizes=1,1
  Selector14 : Selector  NumberOfDimensions=2  InputPortWidth=4  IndexOptions=Select all,Index vector (dialog)  Indices=[1 2],[1 2]  OutputSizes=1,1
  Selector15 : Selector  NumberOfDimensions=2  InputPortWidth=4  IndexOptions=Select all,Index vector (dialog)  Indices=[1 2],[1 2]  OutputSizes=1,1
  Selector5 : Selector  NumberOfDimensions=2  InputPortWidth=4  IndexOptions=Select all,Index vector (dialog)  Indices=[1 2],[3 4]  OutputSizes=1,1
  Selector6 : Selector  NumberOfDimensions=2  InputPortWidth=4  IndexOptions=Select all,Index vector (dialog)  Indices=[1 2],[3 4]  OutputSizes=1,1
  Selector7 : Selector  NumberOfDimensions=2  InputPortWidth=4  IndexOptions=Select all,Index vector (dialog)  Indices=[1 2],[3 4]  OutputSizes=1,1
  Terminator{,1..9} (10 alike) : Terminator
  VehF [3x4] : Outport
  VehM [3x4] : Outport  Port=2
  WhlF [3x4] : Outport  Port=3
  WhlV [3x4] : Outport  Port=4
  WhlAng [3x4] : Outport  Port=5
  SuspH [1x4] : Outport  Port=6
  wires:
  WhlFy [1x4]/1 -> Bus Creator/5  "WhlFy"
  Bus Selector4/1 -> Selector/1  "<WhlPz>"
  Bus Selector4/5 -> Selector4/1  "<WhlFy>"
  WhlFx [1x4]/1 -> Bus Creator/4  "WhlFx"
  WhlPz [1x4]/1 -> Bus Creator/1  "WhlPz"
  Bus Selector4/2 -> Selector1/1  "<WhlRe>"
  VehP [3x4]/1 -> Bus Creator1/1  "VehP"
  Bus Selector3/1 -> Selector6/1  "<VehP>"
  WhlM [3x4]/1 -> Bus Creator/6  "WhlM"
  Bus Selector4/6 -> Selector5/1  "<WhlM>"
  Bus Selector3/2 -> Selector7/1  "<VehV>"
  WhlVz [1x4]/1 -> Bus Creator/3  "WhlVz"
  Bus Selector4/4 -> Selector3/1  "<WhlFx>"
  VehV [3x4]/1 -> Bus Creator1/2  "VehV"
  WhlRe [1x4]/1 -> Bus Creator/2  "WhlRe"
  Bus Selector4/3 -> Selector2/1  "<WhlVz>"
  Bus Selector1/3 -> Selector10/1  "<WhlVz>"
  Bus Selector1/4 -> Selector11/1  "<WhlFx>"
  Bus Selector2/2 -> Selector15/1  "<VehV>"
  Bus Selector1/6 -> Selector13/1  "<WhlM>"
  Bus Selector2/1 -> Selector14/1  "<VehP>"
  Bus Selector1/2 -> Selector9/1  "<WhlRe>"
  Bus Selector1/5 -> Selector12/1  "<WhlFy>"
  Bus Selector1/1 -> Selector8/1  "<WhlPz>"
  Bus Creator/1 -> Bus Selector4/1, Bus Selector1/1
  StrgAngF [1x2]/1 -> Independent Suspension - Double Wishbone FrontAxle/9  "SrtgAngF"
  Bus Creator1/1 -> Bus Selector2/1, Bus Selector3/1
  Independent Suspension - Double Wishbone FrontAxle/2 -> Terminator/1
  Independent Suspension - Double Wishbone FrontAxle/3 -> Terminator1/1
  Independent Suspension - Double Wishbone FrontAxle/4 -> Terminator2/1
  Independent Suspension - Double Wishbone FrontAxle/5 -> Terminator3/1
  Independent Suspension - Double Wishbone FrontAxle/6 -> Terminator4/1
  Independent Suspension - Double Wishbone RearAxle/2 -> Terminator5/1
  Independent Suspension - Double Wishbone RearAxle/3 -> Terminator6/1
  Independent Suspension - Double Wishbone RearAxle/4 -> Terminator7/1
  Independent Suspension - Double Wishbone RearAxle/5 -> Terminator8/1
  Independent Suspension - Double Wishbone RearAxle/6 -> Terminator9/1
  Rearrange Signals/4(WhlV) -> WhlV [3x4]/1
  Rearrange Signals/2(VehM) -> VehM [3x4]/1
  Rearrange Signals/3(WhlF) -> WhlF [3x4]/1
  Rearrange Signals/5(WhlAng) -> WhlAng [3x4]/1
  Rearrange Signals/1(VehF) -> VehF [3x4]/1
  Rearrange Signals/6(SuspH) -> SuspH [1x4]/1
  Independent Suspension - Double Wishbone FrontAxle/1 -> Rearrange Signals/1(Info f)  "Info f"
  Independent Suspension - Double Wishbone RearAxle/1 -> Rearrange Signals/2(Info r)  "Info r"
  Selector8/1 -> Independent Suspension - Double Wishbone FrontAxle/1
  Selector9/1 -> Independent Suspension - Double Wishbone FrontAxle/2
  Selector10/1 -> Independent Suspension - Double Wishbone FrontAxle/3
  Selector11/1 -> Independent Suspension - Double Wishbone FrontAxle/4
  Selector12/1 -> Independent Suspension - Double Wishbone FrontAxle/5
  Selector13/1 -> Independent Suspension - Double Wishbone FrontAxle/6
  Selector14/1 -> Independent Suspension - Double Wishbone FrontAxle/7
  Selector15/1 -> Independent Suspension - Double Wishbone FrontAxle/8
  Selector/1 -> Independent Suspension - Double Wishbone RearAxle/1
  Selector1/1 -> Independent Suspension - Double Wishbone RearAxle/2
  Selector2/1 -> Independent Suspension - Double Wishbone RearAxle/3
  Selector3/1 -> Independent Suspension - Double Wishbone RearAxle/4
  Selector4/1 -> Independent Suspension - Double Wishbone RearAxle/5
  Selector5/1 -> Independent Suspension - Double Wishbone RearAxle/6
  Selector6/1 -> Independent Suspension - Double Wishbone RearAxle/7
  Selector7/1 -> Independent Suspension - Double Wishbone RearAxle/8

== system nonlineardtm/Nonlinear Dual Track Model/Vehicle Body ==
  FExt [3x1] : Inport
  MExt [3x1] : Inport  Port=2
  WindXYZ [3x1] : Inport  Port=3
  FSusp [3x4] : Inport  Port=4
  MSusp [3x4] : Inport  Port=5
  Terminator{,1..5} (6 alike) : Terminator
  Vehicle Body 6DOF - TUM : vehdynlibeom_TUM/Vehicle Body 6DOF  m=VEH__VehicleData__m_Vehicle_kg  a=VEH__VehicleData__l_WheelbaseF_m  b=VEH__VehicleData__l_WheelbaseTotal_m - VEH__VehicleData__l_WheelbaseF_m  d=- VEH__VehicleData__w_GeomCenterlineToCOG_m  h=VEH__VehicleData__h_AxlePlaneToCOG_m  Xe0=0  Ye0=0  Ze0=0  vx0_mps=INIT__initialvalues__Vehicle_InitialVelocity_mps__1  vy0_mps=- INIT__initialvalues__Vehicle_InitialVelocity_mps__2  vz0_mps=- INIT__initialvalues__Vehicle_InitialVelocity_mps__3  phi0_rad=INIT__initialvalues__Vehicle_InitialRollAngle  theta0_rad=- INIT__initialvalues__Vehicle_InitialPitchAngle  psi0_rad=- INIT__initialvalues__Vehicle_InitialYawAngle  phidot0_radps=INIT__initialvalues__Vehicle_InitialRollRate_radps  thetadot0_radps=- INIT__initialvalues__Vehicle_InitialPitchRate_radps  psidot0_radps=- INIT__initialvalues__Vehicle_InitialYawRate_radps  Iveh=[VEH__VehicleData__I_K_Vehicle_kgm2__11, VEH__VehicleData__I_K_Vehicle_kgm2__12, VEH__VehicleData__I_K_Vehicle_kgm2__13; VEH__VehicleData__I_K_Vehicle_kgm2__21, VEH__VehicleData__I_K_Vehicle_kgm2__22, VEH__VehicleData__I_K_Vehicle_kgm2__23; VEH__VehicleData__I_K_Vehicle_kgm2__31, VEH__VehicleData__I_K_Vehicle_kgm2__32, VEH__VehicleData__I_K_Vehicle_kgm2__33]  tw_front=VEH__VehicleData__w_TrackF_m  tw_rear=VEH__VehicleData__w_TrackR_m  z1m=0  z1R=[-.25,.125,.15]  z1I=[1.4,-.2,.1;-.2,1.4,.1;.1,.1,2.25].*0  z2m=0  z2R=[1.4,0,.8]  z2I=[1.4,-.2,.1;-.2,1.4,.1;.1,.1,2.25].*0  z3m=0  z3R=[.75,-.5,.4]  z3I=[5,-.1,-2;-2,9,.1;-.1,.1,6].*0  z4m=0  z4R=[.75,.5,.4]  z4I=[5,-.1,-2;-2,9,.1;-.1,.1,6].*0  z5m=0  z5R=[1.25,-.5,.4]  z5I=[5,-.1,-2;-2,9,.1;-.1,.1,6].*0  z6m=0  z6R=[1.25,-.5,.4]  z6I=[5,-.1,-2;-2,9,.1;-.1,.1,6].*0  z7m=0  z7R=[2,0,.25]  z7I=[1.4,-.2,.1;-.2,1.4,.1;.1,.1,2.25].*0  Af=VEH__Aerodynamics__A_LongitudinalDrag_m2  Cd=VEH__Aerodynamics__cw_LongitudinalDrag  Cl=abs(VEH__Aerodynamics__cl_LongitudinalLift)  Cpm=VEH__Aerodynamics__cpm_LongDragPitchMomentCoeff  beta_w=[VEH__Aerodynamics__beta_wind_start_rad:VEH__Aerodynamics__beta_wind_step_rad:VEH__Aerodynamics__beta_wind_end_rad]  Cs=[VEH__Aerodynamics__Cs_LatDragCoeff_start:VEH__Aerodynamics__Cs_LatDragCoeff_step:VEH__Aerodynamics__Cs_LatDragCoeff_end]  Cym=[VEH__Aerodynamics__Cym_DragYawMomentCoeff_start:VEH__Aerodynamics__Cym_DragYawMomentCoeff_step:VEH__Aerodynamics__Cym_DragYawMomentCoeff_end]  sign_cl=sign(VEH__Aerodynamics__cl_LongitudinalLift)  Pabs=VEH__Environment__p_Air_Pa  Tair=VEH__Environment__T_Air_K  g=VEH__Environment__a_Gravity_mps2  xdot_tol=VEH__Simulation__Sim_LongVelTolerance_mps  longOff=VEH__Simulation__Sim_LongOff_m  latOff=VEH__Simulation__Sim_LatOff_m  vertOff=VEH__Simulation__Sim_VertOff_m  aMode=2
  Vehicle Routing : Subsystem
  InertFrm.Cg.Disp [3x1] : Outport
  InertFrm.Cg.Vel [3x1] : Outport  Port=2
  InertFrm.Cg.Ang [3x1] : Outport  Port=3
  InertFrm.Axl.Disp [3x4] : Outport  Port=4
  InertFrm.Axl.Vel [3x4] : Outport  Port=5
  BdyFrm.Cg.Vel [3x1] : Outport  Port=6
  BdyFrm.Cg.AngVel [3x1] : Outport  Port=7
  BdyFrm.Cg.Acc [3x1] : Outport  Port=8
  BdyFrm.Cg.AccRel [3x1] : Outport  Port=9
  BdyFrm.Axl.Disp [3x4] : Outport  Port=10
  BdyFrm.Axl.Vel [3x4] : Outport  Port=11
  BdyFrm.Cg.DCM [3x3] : Outport  Port=12
  BdyFrm.Forces.Grvty [3x1] : Outport  Port=13
  BdyFrm.Forces.Drag [3x1] : Outport  Port=14
  BdyFrm.Moments.Drag [3x1] : Outport  Port=15
  BdyFrm.Forces.Body [3x1] : Outport  Port=16
  BdyFrm.Moments.Body [3x1] : Outport  Port=17
  wires:
  Vehicle Body 6DOF - TUM/2 -> Terminator/1
  Vehicle Body 6DOF - TUM/3 -> Terminator1/1
  Vehicle Body 6DOF - TUM/6 -> Terminator4/1
  Vehicle Body 6DOF - TUM/7 -> Terminator5/1
  FSusp [3x4]/1 -> Vehicle Body 6DOF - TUM/1
  MSusp [3x4]/1 -> Vehicle Body 6DOF - TUM/2
  FExt [3x1]/1 -> Vehicle Body 6DOF - TUM/3
  MExt [3x1]/1 -> Vehicle Body 6DOF - TUM/4
  WindXYZ [3x1]/1 -> Vehicle Body 6DOF - TUM/5
  Vehicle Body 6DOF - TUM/1 -> Vehicle Routing/1(Vehicle Info)
  Vehicle Body 6DOF - TUM/4 -> Terminator2/1
  Vehicle Routing/7(BdyFrm.Cg.AngVel) -> BdyFrm.Cg.AngVel [3x1]/1
  Vehicle Routing/12(BdyFrm.Cg.DCM) -> BdyFrm.Cg.DCM [3x3]/1
  Vehicle Routing/2(InertFrm.Cg.Vel) -> InertFrm.Cg.Vel [3x1]/1
  Vehicle Routing/6(BdyFrm.Cg.Vel) -> BdyFrm.Cg.Vel [3x1]/1
  Vehicle Routing/5(InertFrm.Axl.Vel) -> InertFrm.Axl.Vel [3x4]/1
  Vehicle Routing/1(InertFrm.Cg.Disp) -> InertFrm.Cg.Disp [3x1]/1
  Vehicle Routing/8(BdyFrm.Cg.Acc) -> BdyFrm.Cg.Acc [3x1]/1
  Vehicle Routing/10(BdyFrm.Axl.Disp) -> BdyFrm.Axl.Disp [3x4]/1
  Vehicle Routing/14(BdyFrm.Forces.Drag) -> BdyFrm.Forces.Drag [3x1]/1
  Vehicle Routing/13(BdyFrm.Forces.Grvty) -> BdyFrm.Forces.Grvty [3x1]/1
  Vehicle Routing/11(BdyFrm.Axl.Vel) -> BdyFrm.Axl.Vel [3x4]/1
  Vehicle Routing/15(BdyFrm.Moments.Drag) -> BdyFrm.Moments.Drag [3x1]/1
  Vehicle Routing/16(BdyFrm.Forces.Body) -> BdyFrm.Forces.Body [3x1]/1
  Vehicle Routing/4(InertFrm.Axl.Disp) -> InertFrm.Axl.Disp [3x4]/1
  Vehicle Routing/17(BdyFrm.Moments.Body) -> BdyFrm.Moments.Body [3x1]/1
  Vehicle Routing/9(BdyFrm.Cg.AccRel) -> BdyFrm.Cg.AccRel [3x1]/1
  Vehicle Routing/3(InertFrm.Cg.Ang) -> Terminator3/1
  Vehicle Body 6DOF - TUM/5 -> InertFrm.Cg.Ang [3x1]/1
